simulink model "vx_estimator_base"  (R2024b)
settings: Solver=FixedStepAuto  StartTime=0.0  StopTime=10.0  FixedStep=0.004  RelTol=1e-3
model workspace (MAT data in the model file):
  mbd_rack_movement = [-24.295 -24.2949831878 -24.2949831878 -24.2949831878 -24.2949831877 -24.2949831876 -24.2949831874 -24.2949831869 -24.2949831849 -24.2949831786 -24.2949831545 -24.2949831492 ... (273 elements, 273x1)]
  rack_mm = [-25.136 -25.1276327886 -25.1095284284 -25.0914240682 -25.073319708 -25.0564044471 -25.0415413809 -25.0266783147 -25.0118152486 -24.9987131808 -24.9886873592 -24.9786615375 ... (4070 elements, 4070x1)]
  steer_sensor = [701.530379071 702.453261845 703.675449618 704.897637391 706.119825165 707.135081137 707.617795373 708.10050961 708.583223846 709.091528196 709.761580489 710.431632781 ... (4070 elements, 4070x1)]
  wheel_steer_left = [22.9038666573 22.9079555 22.904490995 22.7859585761 22.785958576 22.7859585758 22.7859585755 22.7859585748 22.7859585724 22.7859585657 22.7859585412 22.7859585359 ... (273 elements, 273x1)]
  wheel_steer_right = [23.2682364009 23.2679586767 23.2681940775 23.3035254873 23.3035254873 23.3035254872 23.3035254871 23.3035254866 23.3035254847 23.3035254783 23.3035254538 23.3035254484 ... (273 elements, 273x1)]
libraries: matrix_library x2, simulink_extras x1, sharedTrackingLibrary x1
(part 2 of 2)

== matlab function vx_estimator_base/MATLAB Function1 ==
  data: rpm_FL input; v_wheels output; rpm_FR input; rpm_RL input; rpm_RR input; tire_radius input; delta_rad input; yawrate_rad_s input; tr input; brake_pedal input; perc_diff output; using_front_vel output
function [v_wheels, perc_diff, using_front_vel] = estimateVx4Wheels(rpm_FL, rpm_FR, rpm_RL, rpm_RR, tire_radius, delta_rad, yawrate_rad_s, tr, brake_pedal)

    gearboxRatio = 11.83;
    
    rads_FL = rpm_FL * 0.10472;
    rads_FR = rpm_FR * 0.10472;

    rads_RL = rpm_RL * 0.10472;
    rads_RR = rpm_RR * 0.10472;
    
    Vx_fl_corner = rads_FL / gearboxRatio * cos(abs(delta_rad)) * tire_radius;
    Vx_fl = Vx_fl_corner - (yawrate_rad_s * (tr/2));
    
    Vx_fr_corner = rads_FR / gearboxRatio * cos(abs(delta_rad)) * tire_radius;
    Vx_fr = Vx_fr_corner + (yawrate_rad_s * (tr/2));

    Vx_rl_corner = rads_RL / gearboxRatio * tire_radius;
    Vx_rl = Vx_rl_corner - (yawrate_rad_s * (tr/2));
    
    Vx_rr_corner = rads_RR / gearboxRatio * tire_radius;
    Vx_rr = Vx_rr_corner + (yawrate_rad_s * (tr/2));
    

    
    

    if(brake_pedal > .05)
        v_wheels = (Vx_fl + Vx_fr)/2;
        using_front_vel = true
        if((Vx_fl + Vx_fr)/2 > 0)
            perc_diff = abs((Vx_fl - Vx_fr)/2) / ((Vx_fl + Vx_fr)/2) ;
        else
            perc_diff = 0;
        end
        
    else
        v_wheels = (Vx_rl + Vx_rr)/2;
        using_front_vel = false
        if((Vx_rl + Vx_rr)/2 > 0)
            perc_diff = abs((Vx_rl - Vx_rr)/2) / ((Vx_rl + Vx_rr)/2) ;
        else
            perc_diff = 0;
        end
    end
    
end

== matlab function vx_estimator_base/MATLAB Function ==
  data: ins_mode input; ins_noise output; vel_u input; v_wheels input; v_INS input
function ins_noise  = estimateINSNoise(ins_mode, vel_u, v_wheels, v_INS)
%ESTIMATEINSNOISE Summary of this function goes here
%   Detailed explanation goes here

if(ins_mode ==0)
    ins_noise = 100;
elseif(ins_mode==1)
    ins_noise = abs(vel_u)*10;
elseif(ins_mode==2)
    ins_noise = abs(vel_u);
else
    ins_noise = 0.5;
end

if( (v_wheels > 0) & (v_INS < 0))
    ins_noise = 20;
end
end
